simulink model "threephase_simscape"  (R2014a)
settings: Solver=ode15s  StartTime=0.0  StopTime=1
libraries: pe_lib x3, fl_lib x2, nesl_utility x2
settings Model: Creator=scastro  LastModifiedBy=cosorio
settings DataIOCC: SaveTime=off  SignalLoggingName=logsoutSC
settings DebuggingCC: UnderspecifiedInitializationDetection=Classic  SolverPrmCheckMsg=none  MultiTaskDSMMsg=warning  MultiTaskCondExecSysMsg=none
settings RTWCC: IncludeERTFirstTime=on

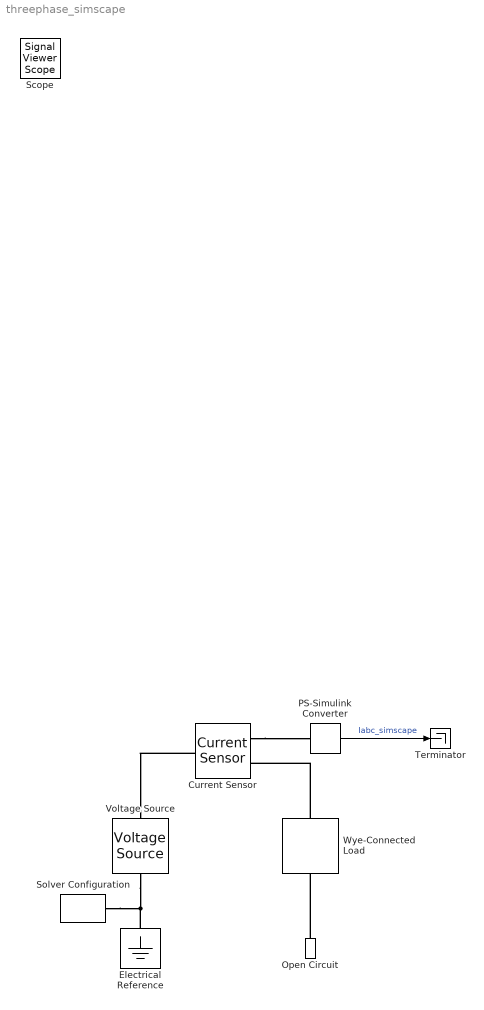
== system threephase_simscape ==
  Current Sensor : pe_lib/Sensors/Current Sensor
  Electrical Reference : fl_lib/Electrical/Electrical Elements/Electrical Reference
  Open Circuit : fl_lib/Electrical/Electrical Elements/Open Circuit
  PS-Simulink Converter : nesl_utility/PS-Simulink Converter  PhysicalDomain=network_engine_domain  SubClassName=ps_output  LeftPortType=input  RightPortType=output  PseudoPeriodic=off  Frequencies=[]  Unit=A  AffineConversion=off
  Solver Configuration : nesl_utility/Solver Configuration  PhysicalDomain=network_engine_domain  SubClassName=solver  LeftPortType=input  RightPortType=generic  Accelerate=off  Tones=[]  Harmonics=[]  SimulateNoise=off  Profile=off  UseLocalSampling=off  EnableSwitchedLinearOptims=on  FrequencyDomain=off  UseCCode=off  RelTol=0.001  AbsTol=1e-06  MinStep=1e-09  ToWorkspace=off  DoDC=off  ResidualTolerance=1e-09  UseLocalSolver=off  LocalSolverChoice=NE_BACKWARD_EULER_ADVANCER  LocalSolverSampleTime=0.001  DoFixedCost=off  MaxNonlinIter=3  MaxModeIter=2  LinearAlgebra=Sparse  DelaysMemoryBudget=1024  AutomaticFiltering=on  FilteringTimeConstant=0.001
  Terminator : Terminator
  Voltage Source : pe_lib/Sources/Voltage Source  vline_rms=sqrt(3) * 100 / sqrt(2) V  shift=0 deg  freq=60 Hz  omega=0 rad/s  shift_3ph=[nan, nan, nan]  sqrt2OverSqrt3=nan
  Wye-Connected Load : pe_lib/Passive Devices/Wye-Connected Load  parameterization=2  component_structure=1  component_structure_PQ=7  R=1 Ohm  L=0.001 H  C=1e-6 F  IL0=[ 0 0 0 ] A  VC0=[ 0 0 0 ] V  R_parasitic=1e-6 Ohm  G_parasitic=1e-6 1/Ohm  VRated=100 V  FRated=60 Hz  P=1000 W  Qpos=100 V*A  Qneg=-100 V*A  Vmag0=100 V  Vang0=0 deg  Freq0=60 Hz  R_parasitic_PQ=1e-6 Ohm  G_parasitic_PQ=1e-6 1/Ohm
  Scope : SignalViewerScope  IOType=viewer  RefreshTime=0.035000
      settings: TimeRange=0.1  YMin=-15  YMax=15
  wires:
  PS-Simulink Converter/1 -> Terminator/1  "Iabc_simscape"
  connections:
  Solver Configuration/RConn1 -- Electrical Reference/LConn1 -- Voltage Source/LConn1
  Current Sensor/RConn1 -- PS-Simulink Converter/LConn1
  Current Sensor/LConn1 -- Voltage Source/RConn1
  Wye-Connected Load/LConn1 -- Current Sensor/RConn2
  Open Circuit/LConn1 -- Wye-Connected Load/RConn1
